simulink model "bf_bioc_new_reg"  (Simulink 6.0)
settings: Solver=ode15s  StartTime=0.0  StopTime=200  MaxStep=10  MinStep=0.0001  RelTol=1e-3  AbsTol=1e-3
settings Model: LastModifiedBy=cgzkn
settings DataIOCC: LimitDataPoints=off

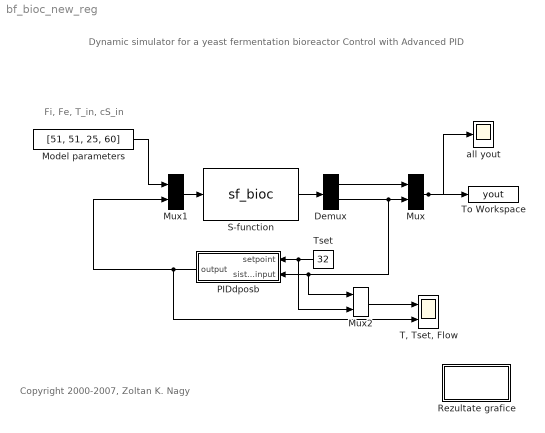
== system bf_bioc_new_reg ==
  note: Dynamic simulator for a yeast fermentation bioreactor
      |
      | Control with Advanced PID
  note: Fi, Fe, T_in, cS_in
  note: Copyright 2000-2007, Zoltan K. Nagy
  Demux : Demux  Outputs=[6 1]
      mask Display: disp('D')
  Model parameters : Constant  Value=[51, 51, 25, 60]
  Mux : Mux  Inputs=[6 1]
      mask Display: disp('M')
  Mux1 : Mux  Inputs=[4 1]
      mask Display: disp('M')
  Mux2 : Mux  Inputs=2
      mask Display: disp('M')
  PIDdposb : Subsystem  Orientation=left  mask(anti windup PID, pos. alg., bckw. aprox){K=5, Ti=10, Td=0, h=0.1}
      mask prompts: K "Factor de amplificare (K)"; Ti "Constanta de integrare (Ti)"; Td "Constanta de derivare (Td)"; h "Constantele : [Tt b inv] (inv= -1 pt sist. inv.)"
      mask help:
      | anti windup PID,
      |  position algoritm,
      |  backward aprox
      |
      | Copyright 2000-2007, Zoltan K. Nagy
      mask init:
      | Tt=@4(1); b=@4(2); inv=@4(3); ulow=@5(1); uhigh=@5(2); ustat=@5(3);
      mask Display: plot(-12,-0.3,4,1.3,[0,1,2,3],[0,0,1,1]);disp('PIDdposb')
  Rezultate grafice : Subsystem
      settings: OpenFcn=bfgraf
      mask Display: disp('Plot\nresults')
  S-function : S-Function  FunctionName=sf_bioc
      mask Display: disp('BIOREACTOR\nMODEL\ncontinuous')
  "T, Tset, Flow" : Scope  NumInputPorts=2
      settings: TimeRange=200  YMin=29.5~2  YMax=32.5~10  DataFormat=Array
  To Workspace : ToWorkspace  VariableName=yout  SaveFormat=Array
  Tset : Constant  Orientation=left  Value=32
  all yout : Scope
      settings: TimeRange=200.000000  YMin=-35  YMax=35  DataFormat=Array
  wires:
  S-function/1 -> Demux/1
  Demux/1 -> Mux/1
  Demux/2 -> Mux/2, PIDdposb/2(sistem  input), Mux2/1
  Mux/1 -> To Workspace/1, all yout/1
  Model parameters/1 -> Mux1/1
  Mux1/1 -> S-function/1
  Tset/1 -> PIDdposb/1(setpoint), Mux2/2
  PIDdposb/1(output) -> Mux1/2, "T, Tset, Flow"/2
  Mux2/1 -> "T, Tset, Flow"/1

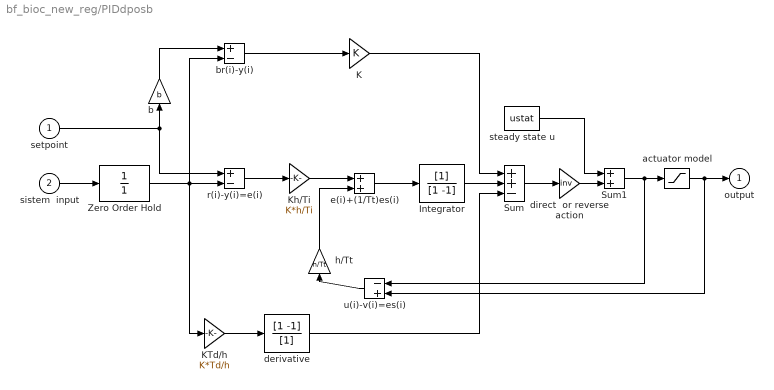
== system bf_bioc_new_reg/PIDdposb ==
  setpoint : Inport  Port=1  LatchInput=off
  sistem  input : Inport  Port=2  LatchInput=off
  Integrator : DiscreteFilter  Denominator=[1 -1]  SampleTime=h
  K : Gain  Gain=K  SaturateOnIntegerOverflow=on
  KTd/h : Gain  Gain=K*Td/h  SaturateOnIntegerOverflow=on
  Kh/Ti : Gain  Gain=K*h/Ti  SaturateOnIntegerOverflow=on
  Sum : Sum  Inputs=++-  SaturateOnIntegerOverflow=on  InputSameDT=on
  Sum1 : Sum  SaturateOnIntegerOverflow=on  InputSameDT=on
  Zero Order Hold : DiscreteTransferFcn  Numerator=1  Denominator=1  SampleTime=h
  actuator model : Saturate  UpperLimit=uhigh  LowerLimit=ulow
  b : Gain  Orientation=up  Gain=b  SaturateOnIntegerOverflow=on
  br(i)-y(i) : Sum  Inputs=+-  SaturateOnIntegerOverflow=on  InputSameDT=on
  derivative : DiscreteFilter  Numerator=[1 -1]  Denominator=[1]  SampleTime=h
  direct  or reverse action : Gain  Gain=inv  SaturateOnIntegerOverflow=on
  e(i)+(1/Tt)es(i) : Sum  SaturateOnIntegerOverflow=on  InputSameDT=on
  h/Tt : Gain  Orientation=up  Gain=h/Tt  SaturateOnIntegerOverflow=on
  r(i)-y(i)=e(i) : Sum  Inputs=+-  SaturateOnIntegerOverflow=on  InputSameDT=on
  steady state u : Constant  Value=ustat
  u(i)-v(i)=es(i) : Sum  Orientation=left  Inputs=-+  SaturateOnIntegerOverflow=on  InputSameDT=on
  output : Outport
  wires:
  setpoint/1 -> b/1, r(i)-y(i)=e(i)/1
  steady state u/1 -> Sum1/1
  actuator model/1 -> output/1, u(i)-v(i)=es(i)/2
  u(i)-v(i)=es(i)/1 -> h/Tt/1
  Sum1/1 -> actuator model/1, u(i)-v(i)=es(i)/1
  derivative/1 -> Sum/3
  KTd/h/1 -> derivative/1
  h/Tt/1 -> e(i)+(1/Tt)es(i)/2
  K/1 -> Sum/1
  br(i)-y(i)/1 -> K/1
  Zero Order Hold/1 -> r(i)-y(i)=e(i)/2, KTd/h/1, br(i)-y(i)/2
  b/1 -> br(i)-y(i)/1
  direct  or reverse action/1 -> Sum1/2
  Sum/1 -> direct  or reverse action/1
  Integrator/1 -> Sum/2
  e(i)+(1/Tt)es(i)/1 -> Integrator/1
  Kh/Ti/1 -> e(i)+(1/Tt)es(i)/1
  r(i)-y(i)=e(i)/1 -> Kh/Ti/1
  sistem  input/1 -> Zero Order Hold/1

== system bf_bioc_new_reg/Rezultate grafice ==
